simulink model "CuantUnifVoz"  (R2013a)
settings: Solver=VariableStepDiscrete  StartTime=0.0  StopTime=1  RelTol=1e-3
values from neighbouring files (symbols this model uses):
  fs = 1/(tout(2)-tout(1))    [CuantNoUniformeVoz.m]    (also in CuantUniformeSeno.m; CuantUniformeVoz.m)
  n = N(i)    [CuantNoUniformeVoz.m]    (also in CuantUniformeSeno.m; CuantUniformeVoz.m)
settings Model: Creator=Jorge Armando  LastModifiedBy=user
settings DataIOCC: LimitDataPoints=off  SignalLoggingSaveFormat=ModelDataLogs
settings DebuggingCC: MultiTaskDSMMsg=warning  MultiTaskCondExecSysMsg=none  StrictBusMsg=None
settings RTWCC: IncludeERTFirstTime=on
settings GRTTargetCC: CodeReplacementLibrary=None  CPPClassGenCompliant=on

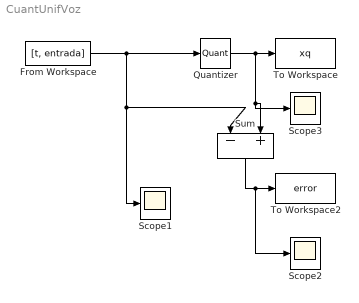
== system CuantUnifVoz ==
  From Workspace : FromWorkspace  VariableName=[t, entrada]  OutDataTypeStr=double  SampleTime=1/fs
  Quantizer : Quantizer  QuantizationInterval=1.14*2^(-n)
  Scope1 : Scope
  Scope2 : Scope
      settings: SaveName=ScopeData2
  Scope3 : Scope
      settings: SaveName=ScopeData3
  Sum : Sum  Inputs=|-+
  To Workspace : ToWorkspace  VariableName=xq  SampleTime=-1
  To Workspace2 : ToWorkspace  VariableName=error  SampleTime=-1
  wires:
  Quantizer/1 -> Scope3/1, Sum/2, To Workspace/1
  Sum/1 -> Scope2/1, To Workspace2/1
  From Workspace/1 -> Sum/1, Scope1/1, Quantizer/1
